simulink subsystem "diagnostics_2024"  (R2024b)
settings: Solver=VariableStepAuto  StartTime=0.0  StopTime=10.0  RelTol=1e-3
settings Model: Creator=HP ELITEBOOK  LastModifiedBy=HP ELITEBOOK

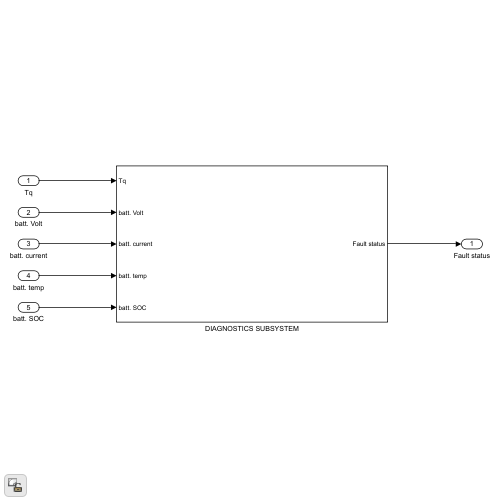
[thumbnail: Simulink's stored preview of the top-level diagram]
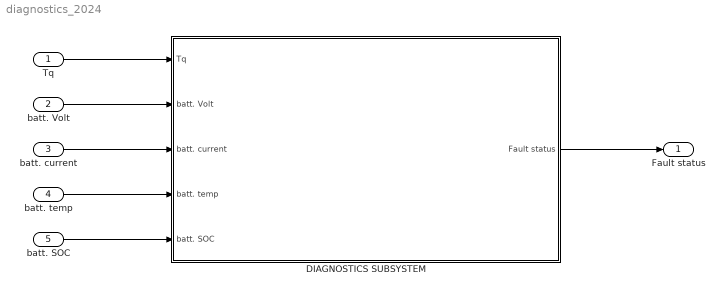
== system diagnostics_2024 ==
  Tq : Inport
  batt. Volt : Inport  Port=2
  batt. current : Inport  Port=3
  batt. temp : Inport  Port=4
  batt. SOC : Inport  Port=5
  DIAGNOSTICS SUBSYSTEM : Subsystem
  Fault status : Outport
  wires:
  Tq/1 -> DIAGNOSTICS SUBSYSTEM/1(Tq)
  batt. Volt/1 -> DIAGNOSTICS SUBSYSTEM/2(batt. Volt)
  batt. current/1 -> DIAGNOSTICS SUBSYSTEM/3(batt. current)
  batt. temp/1 -> DIAGNOSTICS SUBSYSTEM/4(batt. temp)
  batt. SOC/1 -> DIAGNOSTICS SUBSYSTEM/5(batt. SOC)
  DIAGNOSTICS SUBSYSTEM/1(Fault status) -> Fault status/1

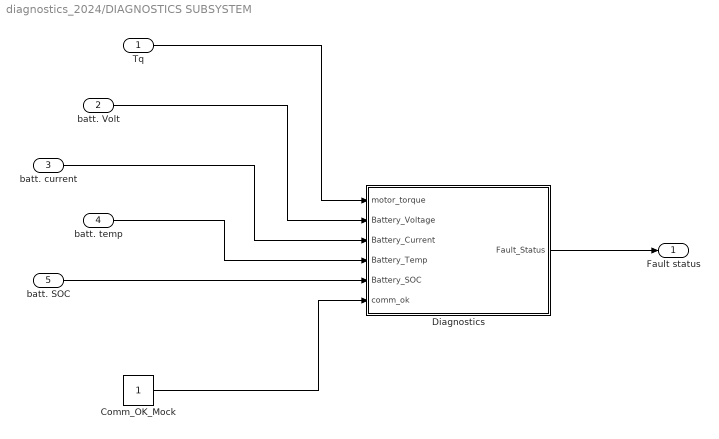
== system diagnostics_2024/DIAGNOSTICS SUBSYSTEM ==
  Tq : Inport
  batt. Volt : Inport  Port=2
  batt. current : Inport  Port=3
  batt. temp : Inport  Port=4
  batt. SOC : Inport  Port=5
  Comm_OK_Mock : Constant
  Diagnostics : Subsystem
  Fault status : Outport
  wires:
  Diagnostics/1(Fault_Status) -> Fault status/1
  batt. temp/1 -> Diagnostics/4(Battery_Temp)
  batt. Volt/1 -> Diagnostics/2(Battery_Voltage)
  batt. current/1 -> Diagnostics/3(Battery_Current)
  Tq/1 -> Diagnostics/1(motor_torque)
  batt. SOC/1 -> Diagnostics/5(Battery_SOC)
  Comm_OK_Mock/1 -> Diagnostics/6(comm_ok)

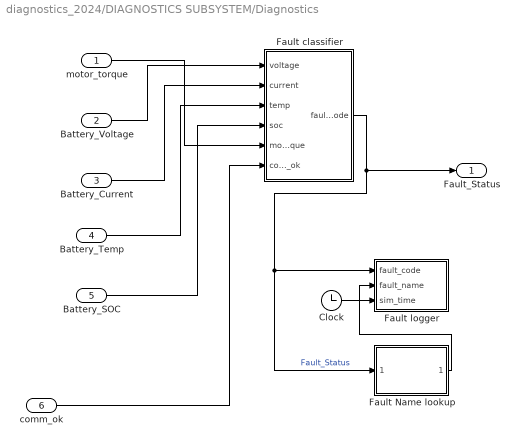
== system diagnostics_2024/DIAGNOSTICS SUBSYSTEM/Diagnostics ==
  motor_torque : Inport
  Battery_Voltage : Inport  Port=2
  Battery_Current : Inport  Port=3
  Battery_Temp : Inport  Port=4
  Battery_SOC : Inport  Port=5
  comm_ok : Inport  Port=6
  Clock : Clock
  Fault Name lookup : MATLAB Function  TreatAsAtomicUnit=on
  Fault classifier : MATLAB Function  TreatAsAtomicUnit=on
  Fault logger : MATLAB Function  TreatAsAtomicUnit=on
  Fault_Status : Outport
  wires:
  comm_ok/1 -> Fault classifier/6(comm_ok)
  Fault Name lookup/1(fault_name) -> Fault logger/2(fault_name)
  Battery_SOC/1 -> Fault classifier/4(soc)
  Clock/1 -> Fault logger/3(sim_time)
  Fault classifier/1(fault_code) -> Fault_Status/1, Fault Name lookup/1(fault_code), Fault logger/1(fault_code)  "Fault_Status"
  Battery_Current/1 -> Fault classifier/2(current)
  Battery_Temp/1 -> Fault classifier/3(temp)
  Battery_Voltage/1 -> Fault classifier/1(voltage)
  motor_torque/1 -> Fault classifier/5(motor_torque)

== matlab function diagnostics_2024/DIAGNOSTICS SUBSYSTEM/Diagnostics/Fault logger ==
  data: fault_code input; fault_name input; sim_time input
function log_fault(fault_code, fault_name, sim_time)

persistent last_code
if isempty(last_code)
    last_code = -1;
end

if fault_code ~= last_code
    fid = fopen('fault_log.csv', 'a');
    if fid ~= -1
        fprintf(fid, '%.3f,%.0f,%s\n', sim_time, fault_code, char(fault_name));
        fclose(fid);
    end
    last_code = fault_code;
end

== matlab function diagnostics_2024/DIAGNOSTICS SUBSYSTEM/Diagnostics/Fault classifier ==
  data: voltage input; fault_code output; current input; temp input; soc input; motor_torque input; comm_ok input
function fault_code = Fault_Classifier(voltage, current, temp, soc, motor_torque, comm_ok)

persistent state
if isempty(state)
    state = 0; % 0 = Normal
end

if voltage > 58
    state = 1; % F001 Critical - overvoltage
elseif state == 1 && voltage < 55
    state = 0;
end

if temp > 45
    state = 2; % F002 Warning - overtemp
elseif state == 2 && temp < 40
    state = 0;
end

if soc < 5
    state = 3; % F003 Critical - low SOC
elseif state == 3 && soc > 10
    state = 0;
end

if motor_torque > 30
    state = 4; % F004 Warning - overtorque
elseif state == 4 && motor_torque < 25
    state = 0;
end

if comm_ok == 0
    state = 5; % F005 Critical - comms lost
elseif state == 5 && comm_ok == 1
    state = 0;
end

if current > 20
    state = 6; % F006 Critical - overcurrent
elseif state == 6 && current < 17
    state = 0;
end

if voltage < 44
    state = 7; % F007 Critical - undervoltage
elseif state == 7 && voltage > 46
    state = 0;
end

fault_code = state;

== matlab function diagnostics_2024/DIAGNOSTICS SUBSYSTEM/Diagnostics/Fault Name lookup ==
  data: fault_code input; fault_name output
function fault_name = Fault_Name_Lookup(fault_code)

switch fault_code
    case 0
        raw = 'NORMAL              ';
    case 1
        raw = 'F001 OVERVOLTAGE    ';
    case 2
        raw = 'F002 OVERTEMP       ';
    case 3
        raw = 'F003 LOW SOC        ';
    case 4
        raw = 'F004 OVERTORQUE     ';
    case 5
        raw = 'F005 COMMS LOST     ';
    case 6
        raw = 'F006 OVERCURRENT    ';
    case 7
        raw = 'F007 UNDERVOLTAGE   ';
    otherwise
        raw = 'UNKNOWN FAULT       ';
end

fault_name = uint8(raw);
